simulink model "dlb_sm22022b"  (R2022b)
settings: Solver=FixedStepAuto  StartTime=0.0  StopTime=10.0  FixedStep=1e-6  RelTol=1e-3
settings Model: Creator=Zenos  LastModifiedBy=Zenos
settings OptimizationCC: ReuseModelBlockBuffer=on

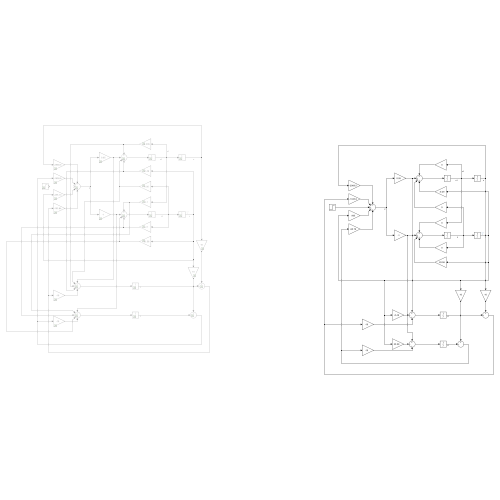
[thumbnail: Simulink's stored preview of the top-level diagram]
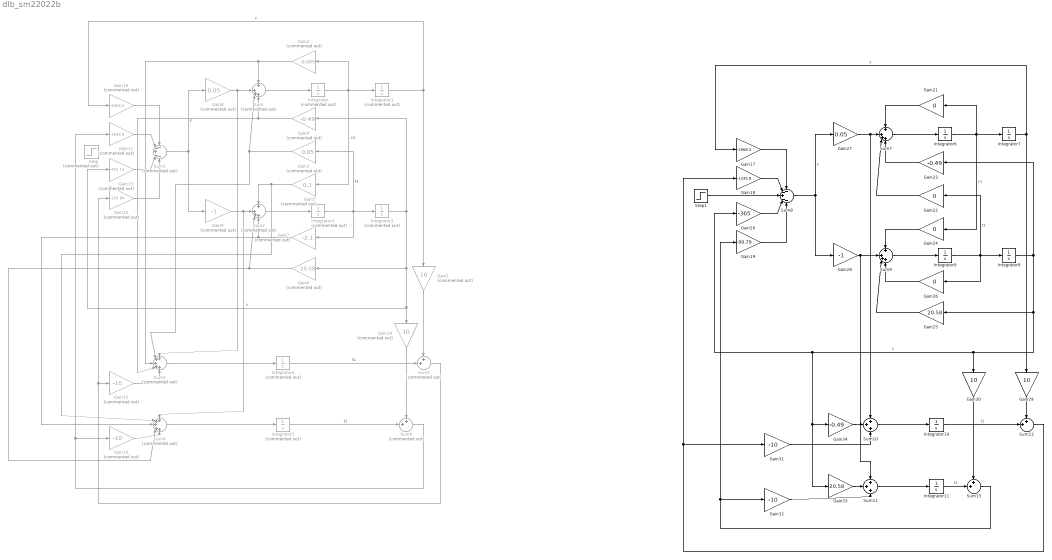
== system dlb_sm22022b ==
  Gain1 : Gain  Commented=on  Gain=10
  Gain10 : Gain  Commented=on  Gain=-2968.5
  Gain11 : Gain  Commented=on  Gain=-1638.8
  Gain12 : Gain  Commented=on  Gain=-103.84
  Gain13 : Gain  Commented=on  Gain=-455.13
  Gain14 : Gain  Commented=on  Gain=10
  Gain15 : Gain  Commented=on  Gain=-10
  Gain16 : Gain  Commented=on  Gain=-10
  Gain17 : Gain  Gain=-2968.5
  Gain18 : Gain  Gain=-1335.8
  Gain19 : Gain  Gain=-90.79
  Gain2 : Gain  Commented=on  Gain=-0.005
  Gain20 : Gain  Gain=-365
  Gain{21..22,24,26} (4 alike) : Gain  Gain=0
  Gain23 : Gain  Gain=-0.49
  Gain25 : Gain  Gain=20.58
  Gain27 : Gain  Gain=0.05
  Gain28 : Gain  Gain=-1
  Gain29 : Gain  Gain=10
  Gain3 : Gain  Commented=on  Gain=0.05
  Gain30 : Gain  Gain=10
  Gain31 : Gain  Gain=-10
  Gain32 : Gain  Gain=-10
  Gain33 : Gain  Gain=20.58
  Gain34 : Gain  Gain=-0.49
  Gain4 : Gain  Commented=on  Gain=-0.49
  Gain5 : Gain  Commented=on  Gain=0.1
  Gain6 : Gain  Commented=on  Gain=20.58
  Gain7 : Gain  Commented=on  Gain=-2.1
  Gain8 : Gain  Commented=on  Gain=0.05
  Gain9 : Gain  Commented=on  Gain=-1
  Integrator{,1,3..5} (5 alike) : Integrator  Commented=on
  Integrator{6..7,9..11} (5 alike) : Integrator
  Integrator2 : Integrator  Commented=on  InitialCondition=-1
  Integrator8 : Integrator  InitialCondition=-1
  Step : Step  Commented=on  After=1000  SampleTime=0
  Step1 : Step  After=1000  SampleTime=0
  Sum : Sum  Commented=on  Inputs=+|+++
  Sum1 : Sum  Commented=on  Inputs=--+--
  Sum10 : Sum  Inputs=+++
  Sum11 : Sum  Inputs=+++
  Sum12 : Sum  Inputs=++|
  Sum13 : Sum  Inputs=++|
  Sum2 : Sum  Commented=on  Inputs=+|+++
  Sum3 : Sum  Commented=on  Inputs=+++++
  Sum4 : Sum  Commented=on  Inputs=+++++
  Sum5 : Sum  Commented=on  Inputs=++|
  Sum6 : Sum  Commented=on  Inputs=++|
  Sum7 : Sum  Inputs=+|+++
  Sum8 : Sum  Inputs=--+--
  Sum9 : Sum  Inputs=+|+++
  wires:
  Gain6/1 -> Sum4/4, Sum2/3
  Gain12/1 -> Sum1/5
  Gain11/1 -> Sum1/2
  Gain8/1 -> Sum3/1, Sum/2
  Gain10/1 -> Sum1/1
  Gain9/1 -> Sum2/2, Sum4/1
  Sum/1 -> Integrator/1
  Integrator/1 -> Gain2/1, Gain5/1, Integrator1/1  "x1"
  Sum1/1 -> Gain9/1, Gain8/1  "F"
  Integrator1/1 -> Gain1/1, Gain10/1  "x"
  Gain5/1 -> Sum2/1, Sum4/2
  Gain7/1 -> Sum4/3, Sum2/4
  Integrator2/1 -> Gain6/1, Gain14/1, Gain13/1, Gain4/1  "t"
  Gain13/1 -> Sum1/4
  Gain4/1 -> Sum3/4, Sum/4
  Sum2/1 -> Integrator3/1
  Integrator3/1 -> Gain7/1, Integrator2/1, Gain3/1  "t1"
  Gain3/1 -> Sum3/2, Sum/3
  Gain2/1 -> Sum/1, Sum3/3
  Sum3/1 -> Integrator4/1
  Sum4/1 -> Integrator5/1
  Gain1/1 -> Sum5/1
  Integrator4/1 -> Sum5/2  "t1"
  Integrator5/1 -> Sum6/2  "t1"
  Gain14/1 -> Sum6/1
  Sum5/1 -> Gain12/1, Gain15/1
  Gain15/1 -> Sum3/5
  Sum6/1 -> Gain11/1, Gain16/1
  Gain16/1 -> Sum4/5
  Sum8/1 -> Gain28/1, Gain27/1  "F"
  Gain22/1 -> Sum7/3
  Gain26/1 -> Sum9/4
  Gain19/1 -> Sum8/5
  Sum9/1 -> Integrator9/1
  Step1/1 -> Sum8/3
  Gain17/1 -> Sum8/1
  Gain27/1 -> Sum7/2, Sum10/1
  Gain25/1 -> Sum9/3
  Gain24/1 -> Sum9/1
  Integrator7/1 -> Gain17/1, Gain29/1  "x"
  Gain20/1 -> Sum8/4
  Gain18/1 -> Sum8/2
  Gain28/1 -> Sum9/2, Sum11/1
  Gain23/1 -> Sum7/4
  Gain21/1 -> Sum7/1
  Sum7/1 -> Integrator6/1
  Integrator8/1 -> Gain25/1, Gain20/1, Gain33/1, Gain34/1, Gain30/1, Gain23/1  "t"
  Integrator9/1 -> Gain26/1, Integrator8/1, Gain22/1  "t1"
  Integrator6/1 -> Gain21/1, Gain24/1, Integrator7/1  "x1"
  Integrator11/1 -> Sum13/2  "t1"
  Sum11/1 -> Integrator11/1
  Sum12/1 -> Gain31/1, Gain18/1
  Integrator10/1 -> Sum12/2  "t1"
  Gain30/1 -> Sum13/1
  Sum13/1 -> Gain32/1, Gain19/1
  Gain29/1 -> Sum12/1
  Sum10/1 -> Integrator10/1
  Gain32/1 -> Sum11/3
  Gain31/1 -> Sum10/3
  Gain33/1 -> Sum11/2
  Gain34/1 -> Sum10/2
